simulink model "MotMapped_EV_Rear"  (R2020a)
settings: configuration reference "Reference" (kept outside this file)
undefined symbols (not defined in the file): w_eff_bp_EV_rear
libraries: autolibmappedmotor x1
settings Model: DataDictionary=System_Data_Dictionary.sldd  ModifiedByFormat=The MathWorks, Inc.  PauseTimes=10  OrderedModelArguments=off  Creator=The MathWorks, Inc.  LastModifiedBy=The MathWorks, Inc.
settings ConfigSetRef: SourceName=Reference

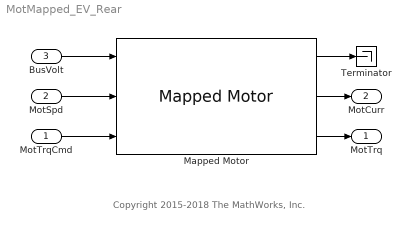
== system MotMapped_EV_Rear ==
  note: Copyright 2015-2018 The MathWorks, Inc.
  MotTrqCmd : Inport
  MotSpd : Inport  Port=2
  BusVolt : Inport  Port=3
  Mapped Motor : autolibmappedmotor/Mapped Motor  port_config=Speed  param_by=Tabulated torque-speed envelope  w_t=w_eff_bp_EV_rear.*pi/30  T_t=T_t_EV_rear  torque_max=torque_max  power_max=power_max  Tc=Tc_Mot  param_loss=Tabulated efficiency data  eff=100  w_eff=375  T_eff=0.08  Piron=0  Pbase=0  w_eff_bp=w_eff_bp_EV_rear.*pi/30  T_eff_bp=T_eff_bp_EV_rear  Temp_eff_bp=[233.15 293.15 373.15]  losses_table=[1 2;3 4]  losses_table_3d=cat(3,1.05*[1.49 1.67 2.21 3.10; 0.42 0.69 1.14 2.03; 0.06 0.24 0.78 1.68; 0.42 0.69 1.14 2.03; 1.49 1.67 2.21 3.10],[1.49 1.67 2.21 3.10; 0.42 0.69 1.14 2.03; 0.06 0.24 0.78 1.68; 0.42 0.69 1.14 2.03; 1.49 1.67 2.21 3.10],1.03*[1.49 1.67 2.21 3.10; 0.42 0.69 1.14 2.03; 0.06 0.24 0.78 1.68; 0.42 0.69 1.14 2.03; 1.49 1.67 2.21 3.10])  efficiency_table=efficiency_table_EV  efficiency_table_3d=cat(3,90*ones(5,4),95*ones(5,4),92*ones(5,4))  J=5e-6  b=1e-5  omega_o=0  T_t_extended=[47.74648293 52.08707228 57.29577951 63.66197724 71.61972439 81.85111359 95.49296586 114.591559 143.2394488 190.9859317 200 200 200 200 200 200 200 190.9859317 143.2394488 114.591559 95.49296586 81.85111359 71.61972439 63.66197724 57.29577951 52.08707228 47.74648293]  w_t_extended=[-2094.3951023932 -1919.86217719376 -1745.32925199433 -1570.7963267949 -1396.26340159546 -1221.73047639603 -1047.1975511966 -872.664625997165 -698.131700797732 -523.598775598299 -499.998830689769 -349.065850398866 -174.532925199433 0 174.532925199433 349.065850398866 499.998830689769 523.598775598299 698.131700797732 872.664625997165 1047.1975511966 1221.73047639603 1396.26340159546 1570.7963267949 1745.32925199433 1919.86217719376 2094.3951023932]  KLossIron=0  KLossCopper=0  x_w_eff_vec=[-2094.3951023932 -1919.86217719376 -1745.32925199433 -1570.7963267949 -1396.26340159546 -1221.73047639603 -1047.1975511966 -872.664625997165 -698.131700797732 -523.598775598299 -499.998830689769 -349.065850398866 -174.532925199433 0 174.532925199433 349.065850398866 499.998830689769 523.598775598299 698.131700797732 872.664625997165 1047.1975511966 1221.73047639603 1396.26340159546 1570.7963267949 1745.32925199433 1919.86217719376 2094.3951023932]  x_T_eff_vec=[-200 -180 -160 -140 -120 -100 -80 -60 -40 -20 0 20 40 60 80 100 120 140 160 180 200]  x_tmp_eff_vec=[233.15 293.15 373.15]  x_losses_mat=[31528.5284231233 28375.675580811 25222.8227384987 22069.9698961863 18917.117053874 15764.2642115617 12611.4113692493 10927.2787950949 9308.4226773031 7391.98271432893 0 6283.18530717959 8377.58040957278 10053.0964914873 11728.6125734019 14660.7657167524 17592.9188601028 20525.0720034533 23457.2251468038 26389.3782901542 29321.5314335047;28901.1510545297 26011.0359490768 23120.9208436238 20230.8057381708 17340.6906327178 14450.5755272649 11560.4604218119 10016.672228837 8532.72078752784 6775.98415480151 0 5759.58653158129 7679.44870877505 9215.33845053005 10751.2281922851 13439.0352403563 16126.8422884276 18814.6493364989 21502.4563845701 24190.2634326414 26878.0704807127;26273.7736859361 23646.3963173425 21019.0189487489 18391.6415801553 15764.2642115617 13136.8868429681 10509.5094743744 9106.06566257911 7757.01889775258 6159.98559527411 0 5235.98775598299 6981.31700797732 8377.58040957278 9773.84381116824 12217.3047639603 14660.7657167524 17104.2266695444 19547.6876223365 21991.1485751285 24434.6095279206;23646.3963173425 21281.7566856083 18917.117053874 16552.4774221398 14187.8377904055 11823.1981586713 9458.558526937 8195.45909632119 6981.31700797732 5543.9870357467 0 4712.38898038469 6283.18530717958 7539.8223686155 8796.45943005141 10995.5742875643 13194.6891450771 15393.80400259 17592.9188601028 19792.0337176157 21991.1485751285;17824.6391693038 16042.1752523734 14259.711335443 12477.2474185127 10694.7835015823 8912.31958465189 7129.85566772151 5347.39175079114 4203.80378974978 4927.98847621928 0 4188.79020478639 3909.5375244673 5026.54824574366 6702.06432765822 8377.58040957277 10053.0964914873 11728.6125734019 13404.1286553164 15079.644737231 16755.1608191455;12860.3208041687 11574.2887237519 10288.256643335 9002.22456291811 7716.19248250124 6430.16040208436 5144.12832166749 4678.96778194224 3678.32831603106 4311.98991669187 0 3665.19142918809 3420.84533390888 4398.22971502571 4886.92190558412 6108.65238198015 7330.38285837617 8552.1133347722 9773.84381116823 10995.5742875643 12217.3047639603;11023.1321178589 9920.81890607302 8818.50569428713 7716.19248250124 6613.87927071535 5511.56605892946 4409.25284714356 4010.54381309335 3152.85284231233 3695.99135716446 0 3141.59265358979 2932.15314335047 3769.91118430775 4188.79020478639 5235.98775598298 6283.18530717958 7330.38285837618 8377.58040957277 9424.77796076937 10471.975511966;9185.94343154909 8267.34908839418 7348.75474523927 6430.16040208437 5511.56605892946 4592.97171577455 4456.15979232595 3342.11984424446 2627.37736859361 3079.99279763705 0 2617.99387799149 2443.46095279206 3141.59265358979 4188.79020478639 4363.32312998582 5235.98775598298 6108.65238198015 6981.31700797731 7853.98163397447 8726.64625997164;7348.75474523927 6613.87927071535 5879.00379619142 5144.12832166749 4409.25284714356 3674.37737261964 3564.92783386076 2673.69587539557 2101.90189487489 2463.99423810964 0 2094.3951023932 1954.76876223365 2513.27412287183 3351.03216382911 3490.65850398865 4188.79020478639 4886.92190558412 5585.05360638185 6283.18530717958 6981.31700797731;6684.23968848892 6015.81571964003 5347.39175079114 4678.96778194224 4010.54381309335 3342.11984424446 2673.69587539557 2005.27190654668 1576.42642115617 1847.99567858223 0 1570.7963267949 1466.07657167524 1884.95559215387 2513.27412287183 3141.59265358979 3769.91118430775 4398.22971502571 5026.54824574366 5654.86677646162 6283.18530717958;8695.63183808294 7826.06865427464 6956.50547046635 5268.80488253735 4516.1184707463 3763.43205895525 3010.7456471642 2608.68955142488 1739.12636761659 1764.70175537566 0 1499.99649206931 1599.99625820726 2399.99438731089 2799.99345186271 3499.99181482838 4199.99017779406 4899.98854075973 6399.98503282904 7199.98316193267 7999.9812910363;6070.7104417194 5463.63939754746 4856.56835337552 4249.49730920358 3642.42626503164 3035.3552208597 2428.28417668776 1821.21313251582 1214.14208834388 1231.99711905482 0 1047.1975511966 1117.01072127637 1675.51608191456 2234.02144255274 2792.52680319093 ...(+4884 chars)]  x_losses_mat_3d=cat(3,[3.255 2.3205 1.7535 1.5645 1.7535 2.3205 3.255;2.1315 1.197 0.7245 0.441 0.7245 1.197 2.1315;1.764 0.819 0.252 0.063 0.252 0.819 1.764;2.1315 1.197 0.7245 0.441 0.7245 1.197 2.1315;3.255 2.3205 1.7535 1.5645 1.7535 2.3205 3.255],[3.1 2.21 1.67 1.49 1.67 2.21 3.1;2.03 1.14 0.69 0.42 0.69 1.14 2.03;1.68 0.78 0.24 0.06 0.24 0.78 1.68;2.03 1.14 0.69 0.42 0.69 1.14 2.03;3.1 2.21 1.67 1.49 1.67 2.21 3.1],[3.193 2.2763 1.7201 1.5347 1.7201 2.2763 3.193;2.0909 1.1742 0.7107 0.4326 0.7107 1.1742 2.0909;1.7304 0.8034 0.2472 0.0618 0.2472 0.8034 1.7304;2.0909 1.1742 0.7107 0.4326 0.7107 1.1742 2.0909;3.193 2.2763 1.7201 1.5347 1.7201 2.2763 3.193])  CalLossMapData={}  CalLossWithTempMapData={}  aMode=aMode  RefBlkName='autolibmappedmotor/Mapped Motor'
      settings: SourceProductBaseCode=PW,MT,VE,VP
  Terminator : Terminator
  MotTrq : Outport  VectorParamsAs1DForOutWhenUnconnected=off
  MotCurr : Outport  Port=2  VectorParamsAs1DForOutWhenUnconnected=off
  wires:
  MotTrqCmd/1 -> Mapped Motor/3
  BusVolt/1 -> Mapped Motor/1
  MotSpd/1 -> Mapped Motor/2
  Mapped Motor/3 -> MotTrq/1
  Mapped Motor/2 -> MotCurr/1
  Mapped Motor/1 -> Terminator/1
